simulink subsystem "sensorLib"  (R2020b)
settings: Solver=VariableStepAuto  StartTime=0.0  StopTime=10.0  RelTol=1e-3
undefined symbols (not defined in the file): States
libraries: sharedtransform x1, mspsensorlib x1
settings Model: Creator=dbell44  LastModifiedBy=dbell44

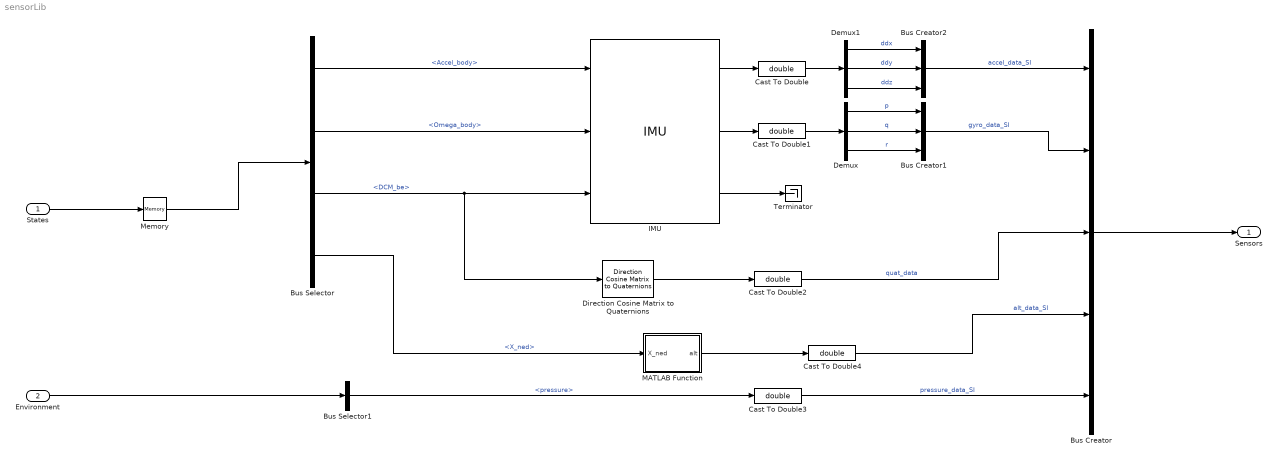
== system sensorLib ==
  States : Inport  OutDataTypeStr=Bus: StatesBus
  Environment : Inport  Port=2  OutDataTypeStr=Bus: EnvironmentBus
  Bus Creator : BusCreator  Inputs=5  OutDataTypeStr=Bus: SensorBus
  Bus Creator1 : BusCreator  Inputs=3  OutDataTypeStr=Bus: gyro_data_SI
  Bus Creator2 : BusCreator  Inputs=3  OutDataTypeStr=Bus: accel_data_SI
  Bus Selector : BusSelector  OutputSignals=Accel_body,Omega_body,DCM_be,X_ned
  Bus Selector1 : BusSelector  OutputSignals=AtmosphereBus.pressure
  Cast To Double{,1..4} (5 alike) : DataTypeConversion  OutDataTypeStr=double
  Demux : Demux  Outputs=3
  Demux1 : Demux  Outputs=3
  Direction Cosine Matrix to Quaternions : sharedtransform/Direction Cosine Matrix  to Quaternions  aMode=0  action=None  tolerance=eps(2)
      settings: SourceProductBaseCode=AE,PW,MT,UV,VE,VP
  IMU : mspsensorlib/IMU  DispRefFrame=NED  Temperature=25  MagneticFieldNED=[ 27.5550, -2.4169, -16.0849 ]  MagneticFieldENU=[ -2.4169, 27.5550, 16.0849 ]  SeedDouble=67  SimulateUsing=Interpreted execution  AccelParamsMeasurementRange=Inf  AccelParamsResolution=0  AccelParamsConstantBias=[ 0, 0, 0 ]  AccelParamsAxesMisalignment=[ 0, 0, 0 ]  AccelParamsNoiseDensity=[ 0, 0, 0 ]  AccelParamsBiasInstability=[ 0, 0, 0 ]  AccelParamsRandomWalk=[ 0, 0, 0 ]  AccelParamsTemperatureBias=[ 0, 0, 0 ]  AccelParamsTemperatureScaleFactor=[ 0, 0, 0 ]  GyroParamsMeasurementRange=Inf  GyroParamsResolution=0  GyroParamsConstantBias=[ 0, 0, 0 ]  GyroParamsAxesMisalignment=[ 0, 0, 0 ]  GyroParamsAccelerationBias=[ 0, 0, 0 ]  GyroParamsNoiseDensity=[ 0, 0, 0 ]  GyroParamsBiasInstability=[ 0, 0, 0 ]  GyroParamsRandomWalk=[ 0, 0, 0 ]  GyroParamsTemperatureBias=[ 0, 0, 0 ]  GyroParamsTemperatureScaleFactor=[ 0, 0, 0 ]  MagParamsMeasurementRange=Inf  MagParamsResolution=0  MagParamsConstantBias=[ 0, 0, 0 ]  MagParamsAxesMisalignment=[ 0, 0, 0 ]  MagParamsNoiseDensity=[ 0, 0, 0 ]  MagParamsBiasInstability=[ 0, 0, 0 ]  MagParamsRandomWalk=[ 0, 0, 0 ]  MagParamsTemperatureBias=[ 0, 0, 0 ]  MagParamsTemperatureScaleFactor=[ 0, 0, 0 ]
      settings: SourceProductBaseCode=TF,NV
  MATLAB Function : MATLAB Function  TreatAsAtomicUnit=on
  Memory : Memory  InitialCondition=States  InheritSampleTime=on
  Terminator : Terminator
  Sensors : Outport  OutDataTypeStr=Bus: SensorBus
  wires:
  States/1 -> Memory/1
  Bus Selector/1 -> IMU/1  "<Accel_body>"
  Memory/1 -> Bus Selector/1
  Bus Selector/2 -> IMU/2  "<Omega_body>"
  Environment/1 -> Bus Selector1/1
  Bus Selector/3 -> IMU/3, Direction Cosine Matrix to Quaternions/1  "<DCM_be>"
  Bus Selector/4 -> MATLAB Function/1(X_ned)  "<X_ned>"
  IMU/3 -> Terminator/1
  Bus Creator/1 -> Sensors/1
  IMU/1 -> Cast To Double/1
  IMU/2 -> Cast To Double1/1
  Cast To Double1/1 -> Demux/1
  Cast To Double/1 -> Demux1/1
  Demux/1 -> Bus Creator1/1  "p"
  Demux/2 -> Bus Creator1/2  "q"
  Demux/3 -> Bus Creator1/3  "r"
  Demux1/1 -> Bus Creator2/1  "ddx"
  Demux1/2 -> Bus Creator2/2  "ddy"
  Demux1/3 -> Bus Creator2/3  "ddz"
  Bus Creator2/1 -> Bus Creator/1  "accel_data_SI"
  Bus Creator1/1 -> Bus Creator/2  "gyro_data_SI"
  Direction Cosine Matrix to Quaternions/1 -> Cast To Double2/1
  Cast To Double2/1 -> Bus Creator/3  "quat_data"
  Bus Selector1/1 -> Cast To Double3/1  "<pressure>"
  Cast To Double3/1 -> Bus Creator/5  "pressure_data_SI"
  MATLAB Function/1(alt) -> Cast To Double4/1
  Cast To Double4/1 -> Bus Creator/4  "alt_data_SI"

== matlab function sensorLib/MATLAB Function ==
  data: X_ned input; alt output
function alt = getAltitude(X_ned)

alt = Sensors.Altimeter(X_ned);
